simulink model "MPC_noConstraints"  (Simulink 10.3)
settings: Solver=FixedStepDiscrete  StartTime=0.0  StopTime=tsim  FixedStep=Ts  RelTol=1e-3  EnableMultiTasking=on
values from neighbouring files (symbols this model uses):
  C_states = eye(4)    [Razzo27.m]
  D_states = [0; 0; 0; 0]    [Razzo27.m]
  P_MPC = P_d    [Razzo27.m]
  Q_MPC = Q_d    [Razzo27.m]
  R_MPC = R_d    (= 100)    [Razzo27.m]
  SetN = [20 30 90]    [Razzo27.m]
  sysd = c2d(sys,Ts)    [Razzo27.m]
  Ts = 0.5*(T_taglio/2)    [Razzo27.m]
  x0 = [deg2rad(0) deg2rad(-15) 0 200]    [Razzo27.m]
  x_ref = [0 0 0 0]'    [Razzo27.m]
undefined symbols (not defined in the file or in its folder): Klqr_d, MPCnoConstraints
settings Model: Creator=Mirko  LastModifiedBy=dadel  MultithreadedSim=on
settings DataIOCC: LimitDataPoints=on
settings GRTTargetCC: CombineOutputUpdateFcns=on  GRTInterface=off
settings ConfigComp: CovSFcnEnable=off

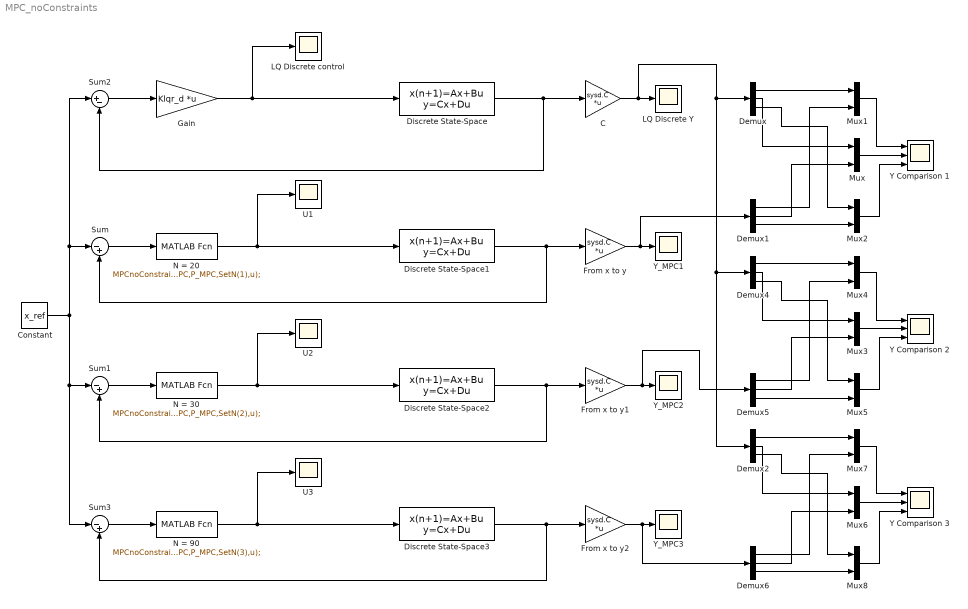
== system MPC_noConstraints ==
  C : Gain  Gain=sysd.C  Multiplication=Matrix(K*u)
  Constant : Constant  Value=x_ref
  Demux{,1..2,4..6} (6 alike) : Demux  Outputs=3
  Discrete State-Space{,1..3} (4 alike) : DiscreteStateSpace  A=sysd.A  B=sysd.B  C=C_states  D=D_states  InitialCondition=x0  SampleTime=Ts
  From x to y : Gain  Gain=sysd.C  Multiplication=Matrix(K*u)
  From x to y1 : Gain  Gain=sysd.C  Multiplication=Matrix(K*u)
  From x to y2 : Gain  Gain=sysd.C  Multiplication=Matrix(K*u)
  Gain : Gain  Gain=Klqr_d  Multiplication=Matrix(K*u)
  LQ Discrete Y : Scope
  LQ Discrete control : Scope
  Mux{,1..8} (9 alike) : Mux  Inputs=2
  N = 20 : MATLABFcn  MATLABFcn=MPCnoConstraints(sysd.A,sysd.B,Q_MPC,R_MPC,P_MPC,SetN(1),u);  OutputDimensions=1
  N = 30 : MATLABFcn  MATLABFcn=MPCnoConstraints(sysd.A,sysd.B,Q_MPC,R_MPC,P_MPC,SetN(2),u);  OutputDimensions=1
  N = 90 : MATLABFcn  MATLABFcn=MPCnoConstraints(sysd.A,sysd.B,Q_MPC,R_MPC,P_MPC,SetN(3),u);  OutputDimensions=1
  Sum : Sum  Inputs=|-+
  Sum1 : Sum  Inputs=|-+
  Sum2 : Sum  Inputs=|+-
  Sum3 : Sum  Inputs=|-+
  U1 : Scope
  U2 : Scope
  U3 : Scope
  Y Comparison 1 : Scope  NumInputPorts=3
  Y Comparison 2 : Scope  NumInputPorts=3
  Y Comparison 3 : Scope  NumInputPorts=3
  Y_MPC1 : Scope
  Y_MPC2 : Scope
  Y_MPC3 : Scope
  wires:
  Discrete State-Space1/1 -> Sum/2, From x to y/1
  Sum/1 -> N = 20/1
  From x to y/1 -> Demux1/1, Y_MPC1/1
  N = 20/1 -> Discrete State-Space1/1, U1/1
  Gain/1 -> Discrete State-Space/1, LQ Discrete control/1
  Sum2/1 -> Gain/1
  Discrete State-Space/1 -> C/1, Sum2/2
  N = 30/1 -> Discrete State-Space2/1, U2/1
  Sum1/1 -> N = 30/1
  Discrete State-Space2/1 -> Sum1/2, From x to y1/1
  N = 90/1 -> Discrete State-Space3/1, U3/1
  Sum3/1 -> N = 90/1
  Discrete State-Space3/1 -> Sum3/2, From x to y2/1
  Demux/1 -> Mux1/1
  Mux1/1 -> Y Comparison 1/1
  Demux1/1 -> Mux1/2
  Demux/2 -> Mux/1
  Demux1/2 -> Mux/2
  Demux1/3 -> Mux2/2
  Demux/3 -> Mux2/1
  Mux2/1 -> Y Comparison 1/3
  Mux/1 -> Y Comparison 1/2
  Demux5/1 -> Mux4/2
  Demux5/2 -> Mux3/2
  Demux4/3 -> Mux5/1
  Demux4/2 -> Mux3/1
  Mux4/1 -> Y Comparison 2/1
  Demux4/1 -> Mux4/1
  Mux5/1 -> Y Comparison 2/3
  C/1 -> Demux2/1, Demux4/1, Demux/1, LQ Discrete Y/1
  Mux3/1 -> Y Comparison 2/2
  Demux5/3 -> Mux5/2
  From x to y1/1 -> Y_MPC2/1, Demux5/1
  Demux2/2 -> Mux6/1
  Demux2/1 -> Mux7/1
  Demux6/2 -> Mux6/2
  From x to y2/1 -> Y_MPC3/1, Demux6/1
  Demux6/3 -> Mux8/2
  Demux6/1 -> Mux7/2
  Demux2/3 -> Mux8/1
  Mux8/1 -> Y Comparison 3/3
  Mux6/1 -> Y Comparison 3/2
  Mux7/1 -> Y Comparison 3/1
  Constant/1 -> Sum3/1, Sum1/1, Sum/1, Sum2/1
